simulink model "control"  (R2020b)
settings: Solver=VariableStepAuto  StartTime=0.0  StopTime=50  RelTol=1e-3
settings Model: Creator=angello  LastModifiedBy=angello

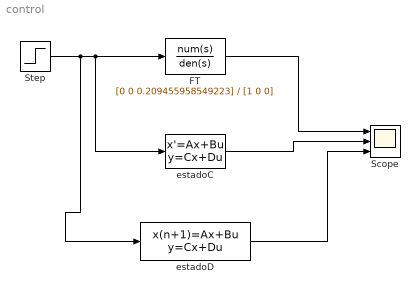
== system control ==
  FT : TransferFcn  Numerator=[0 0 0.209455958549223]  Denominator=[1 0 0]
  Scope : Scope  NumInputPorts=3
  Step : Step  SampleTime=0
  estadoC : StateSpace  A=[0 1;0 0]  B=[0;0.209455958549223]  C=[1 0]  D=0  InitialCondition=0
  estadoD : DiscreteStateSpace  A=[1 0.01;0 1]  B=[1.04727979274611e-05;0.00209455958549223]  C=[1 0]  D=0  SampleTime=0.01
  wires:
  estadoC/1 -> Scope/2
  Step/1 -> estadoD/1, estadoC/1, FT/1
  FT/1 -> Scope/1
  estadoD/1 -> Scope/3
